simulink model "Model"  (R2018b)
settings: Solver=VariableStepAuto  StartTime=0.0  StopTime=400  RelTol=1e-3
values from neighbouring files (symbols this model uses):
  g = 9.81    [MatlabScript1.m]
  J_e = m_c*l_c^2+2*m_p*(l_h^2+l_p^2)    (= 1.054272)    [MatlabScript1.m]
  J_lamda = m_c*l_c^2+2*m_p*l_h^2    (= 1.033536)    [MatlabScript1.m]
  J_p = 2*m_p*l_p^2    (= 0.020736)    [MatlabScript1.m]
  K_de = 10    [MatlabScript1.m]
  K_dp = 10    [MatlabScript1.m]
  K_f = 0.1427    [MatlabScript1.m]
  K_ie = 0.1    [MatlabScript1.m]
  K_ip = 0.1    [MatlabScript1.m]
  K_pe = 1    [MatlabScript1.m]
  K_pp = 1    [MatlabScript1.m]
  l_c = 0.46    [MatlabScript1.m]
  l_h = 0.66    [MatlabScript1.m]
  l_p = 0.12    [MatlabScript1.m]
  m_c = 1.92    [MatlabScript1.m]
  m_p = 0.72    [MatlabScript1.m]
settings Model: Creator=Agurken  LastModifiedBy=Agurken

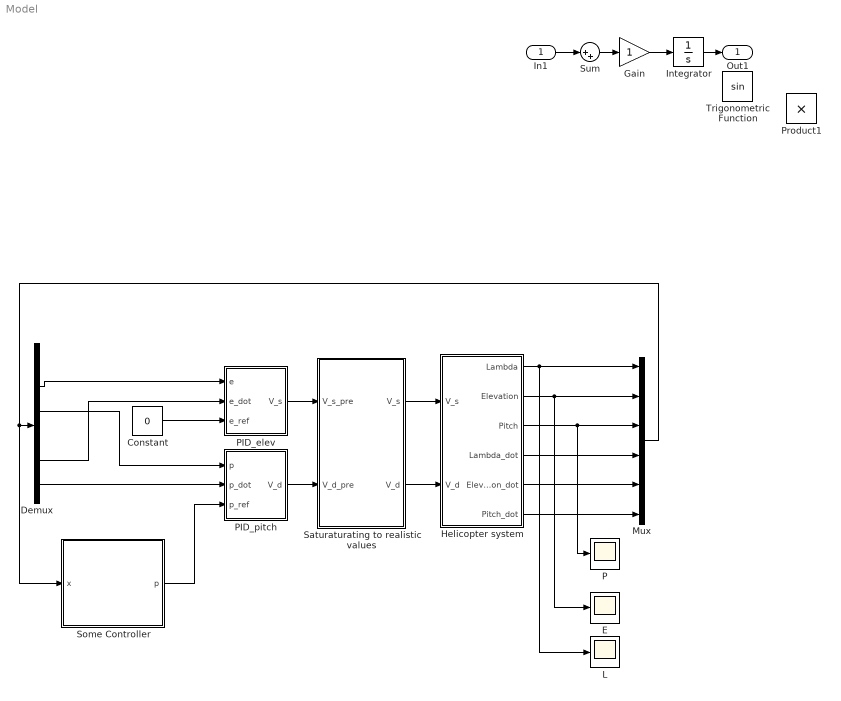
== system Model ==
  In1 : Inport
  Constant : Constant  Value=0  VectorParams1D=off
  Demux : Demux  Outputs=6
  E : Scope
  Gain : Gain
  Helicopter system : Subsystem
  Integrator : Integrator
  L : Scope
  Mux : Mux  Inputs=6
  "P " : Scope
  PID_elev : Subsystem
  PID_pitch : Subsystem
  Product1 : Product
  Saturaturating to realistic values : Subsystem
  Some Controller : Subsystem
  Sum : Sum  Inputs=|++
  Trigonometric Function : Trigonometry
  Out1 : Outport
  wires:
  In1/1 -> Sum/1
  Sum/1 -> Gain/1
  Gain/1 -> Integrator/1
  Integrator/1 -> Out1/1
  Helicopter system/1(Lambda) -> L/1, Mux/1
  Helicopter system/2(Elevation) -> Mux/2, E/1
  Helicopter system/5(Elevation_dot) -> Mux/5
  Constant/1 -> PID_elev/3(e_ref)
  Saturaturating to realistic values/1(V_s) -> Helicopter system/1(V_s)
  PID_elev/1(V_s) -> Saturaturating to realistic values/1(V_s_pre)
  PID_pitch/1("V_d ") -> Saturaturating to realistic values/2(V_d_pre)
  Saturaturating to realistic values/2(V_d) -> Helicopter system/2(V_d)
  Helicopter system/3(Pitch) -> "P "/1, Mux/3
  Helicopter system/4(Lambda_dot) -> Mux/4
  Helicopter system/6(Pitch_dot) -> Mux/6
  Mux/1 -> Some Controller/1(x), Demux/1
  Demux/2 -> PID_elev/1(e)
  Demux/5 -> PID_elev/2(e_dot)
  Demux/3 -> PID_pitch/1(p)
  Demux/6 -> PID_pitch/2(p_dot)
  Some Controller/1(p) -> PID_pitch/3(p_ref)

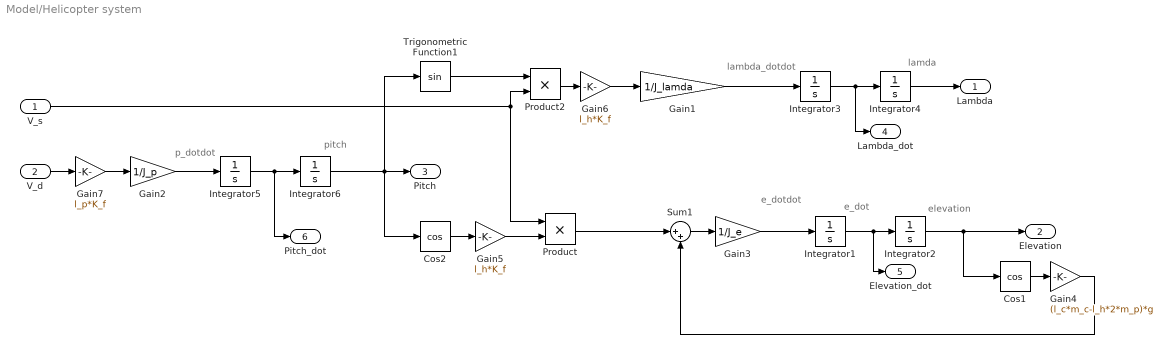
== system Model/Helicopter system ==
  note: elevation
  note: pitch
  note: p_dotdot
  note: lambda_dotdot
  note: lamda
  note: e_dot
  note: e_dotdot
  V_s : Inport
  V_d : Inport  Port=2
  Cos1 : Trigonometry  Operator=cos
  Cos2 : Trigonometry  Operator=cos
  Gain1 : Gain  Gain=1/J_lamda
  Gain2 : Gain  Gain=1/J_p
  Gain3 : Gain  Gain=1/J_e
  Gain4 : Gain  Gain=(l_c*m_c-l_h*2*m_p)*g
  Gain5 : Gain  Gain=l_h*K_f
  Gain6 : Gain  Gain=l_h*K_f
  Gain7 : Gain  Gain=l_p*K_f
  Integrator{1..6} (6 alike) : Integrator
  Product : Product
  Product2 : Product
  Sum1 : Sum  Inputs=|++
  Trigonometric Function1 : Trigonometry
  Lambda : Outport
  Elevation : Outport  Port=2
  Pitch : Outport  Port=3
  Lambda_dot : Outport  Port=4
  Elevation_dot : Outport  Port=5
  Pitch_dot : Outport  Port=6
  wires:
  Gain3/1 -> Integrator1/1
  Integrator2/1 -> Elevation/1, Cos1/1
  Gain1/1 -> Integrator3/1
  Integrator3/1 -> Lambda_dot/1, Integrator4/1
  Product2/1 -> Gain6/1
  V_s/1 -> Product2/2, Product/1
  Gain2/1 -> Integrator5/1
  Gain4/1 -> Sum1/2
  Integrator6/1 -> Pitch/1, Trigonometric Function1/1, Cos2/1
  Sum1/1 -> Gain3/1
  V_d/1 -> Gain7/1
  Gain7/1 -> Gain2/1
  Gain6/1 -> Gain1/1
  Integrator4/1 -> Lambda/1
  Trigonometric Function1/1 -> Product2/1
  Gain5/1 -> Product/2
  Product/1 -> Sum1/1
  Cos2/1 -> Gain5/1
  Cos1/1 -> Gain4/1
  Integrator1/1 -> Elevation_dot/1, Integrator2/1
  Integrator5/1 -> Pitch_dot/1, Integrator6/1

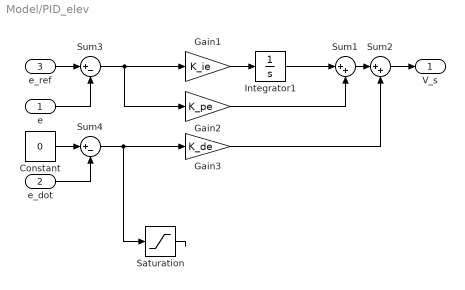
== system Model/PID_elev ==
  e : Inport
  e_dot : Inport  Port=2
  e_ref : Inport  Port=3
  Constant : Constant  Value=0  VectorParams1D=off
  Gain1 : Gain  Gain=K_ie
  Gain2 : Gain  Gain=K_pe
  Gain3 : Gain  Gain=K_de
  Integrator1 : Integrator
  Saturation : Saturate
  Sum1 : Sum  Inputs=|++
  Sum2 : Sum  Inputs=|++
  Sum3 : Sum  Inputs=|+-
  Sum4 : Sum  Inputs=|+-
  V_s : Outport
  wires:
  Gain3/1 -> Sum2/2
  Sum1/1 -> Sum2/1
  Gain1/1 -> Integrator1/1
  Gain2/1 -> Sum1/2
  e_dot/1 -> Sum4/2
  Integrator1/1 -> Sum1/1
  Sum3/1 -> Gain1/1, Gain2/1
  Sum2/1 -> V_s/1
  e/1 -> Sum3/2
  e_ref/1 -> Sum3/1
  Saturation/1 -> ?
  Sum4/1 -> Gain3/1, Saturation/1
  Constant/1 -> Sum4/1

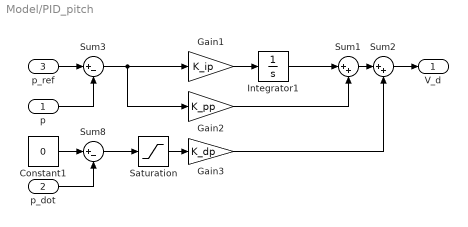
== system Model/PID_pitch ==
  p : Inport
  p_dot : Inport  Port=2
  p_ref : Inport  Port=3
  Constant1 : Constant  Value=0  VectorParams1D=off
  Gain1 : Gain  Gain=K_ip
  Gain2 : Gain  Gain=K_pp
  Gain3 : Gain  Gain=K_dp
  Integrator1 : Integrator
  Saturation : Saturate
  Sum1 : Sum  Inputs=|++
  Sum2 : Sum  Inputs=|++
  Sum3 : Sum  Inputs=|+-
  Sum8 : Sum  Inputs=|+-
  "V_d " : Outport
  wires:
  Gain3/1 -> Sum2/2
  Sum1/1 -> Sum2/1
  Gain1/1 -> Integrator1/1
  Gain2/1 -> Sum1/2
  p_dot/1 -> Sum8/2
  Integrator1/1 -> Sum1/1
  Sum3/1 -> Gain1/1, Gain2/1
  Sum2/1 -> "V_d "/1
  p/1 -> Sum3/2
  p_ref/1 -> Sum3/1
  Saturation/1 -> Gain3/1
  Constant1/1 -> Sum8/1
  Sum8/1 -> Saturation/1

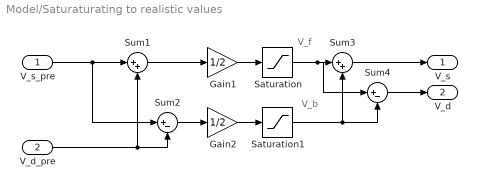
== system Model/Saturaturating to realistic values ==
  note: V_b
  note: V_f
  V_s_pre : Inport
  V_d_pre : Inport  Port=2
  Gain1 : Gain  Gain=1/2
  Gain2 : Gain  Gain=1/2
  Saturation : Saturate  UpperLimit=1000  LowerLimit=0
  Saturation1 : Saturate  UpperLimit=1000  LowerLimit=0
  Sum1 : Sum  Inputs=|++
  Sum2 : Sum  Inputs=|+-
  Sum3 : Sum  Inputs=|++
  Sum4 : Sum  Inputs=|+-
  V_s : Outport
  V_d : Outport  Port=2
  wires:
  V_d_pre/1 -> Sum2/2, Sum1/2
  Saturation1/1 -> Sum4/2, Sum3/2
  Saturation/1 -> Sum4/1, Sum3/1
  Sum4/1 -> V_d/1
  V_s_pre/1 -> Sum2/1, Sum1/1
  Sum1/1 -> Gain1/1
  Sum2/1 -> Gain2/1
  Gain1/1 -> Saturation/1
  Gain2/1 -> Saturation1/1
  Sum3/1 -> V_s/1

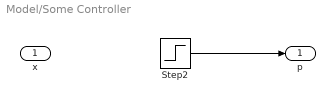
== system Model/Some Controller ==
  x : Inport
  Step2 : Step  Time=20  SampleTime=0
  p : Outport
  wires:
  Step2/1 -> p/1
